simulink model "TemporalEvent"  (R2020b)
settings: Solver=VariableStepAuto  StartTime=0.0  StopTime=10.0  RelTol=1e-3
settings Model: Creator=apple  LastModifiedBy=apple

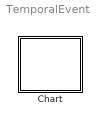
== system TemporalEvent ==
  Chart : Stateflow chart  TreatAsAtomicUnit=on

== stateflow chart TemporalEvent/Chart ==
  state A
    en:fprintf("Entry A");
    du:fprintf("During A");
    ex:fprintf("Exit A");
    state A1
      en:fprintf("Entry A1");
      ex:fprintf("Exit A1");
    (default) -> A1
    (junction 5) -> A1
    A1 -> (junction 5)
  state B
    en:fprintf("Entry B");
    du:fprintf("During B");
    ex:fprintf("Exit B");
  (default) -> A
  A -> B : after(3,E)
  events: E local FUNCTION_CALL_EVENT
